simulink model "ex4"  (R2023b)
settings: Solver=FixedStepDiscrete  StartTime=0.0  StopTime=inf  FixedStep=0.0001  RelTol=1e-3
libraries: simulink_extras x4
settings Model: Creator=Andrei  LastModifiedBy=Andrei

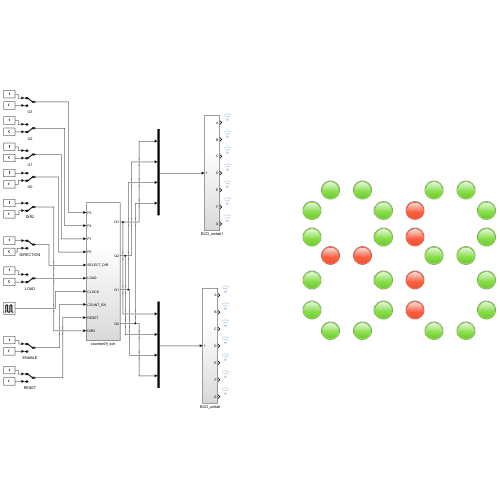
[thumbnail: Simulink's stored preview of the top-level diagram]
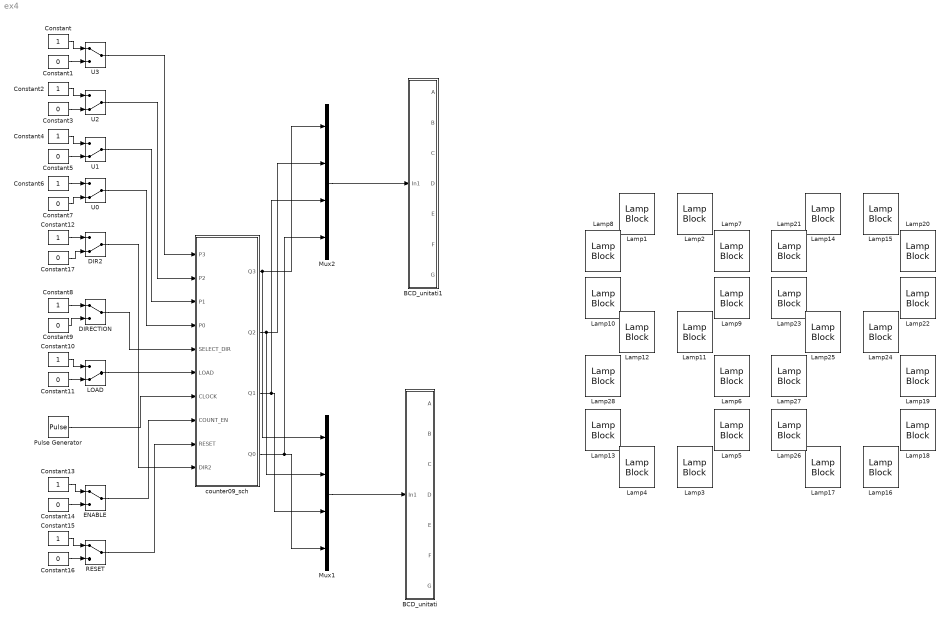
== system ex4 ==
  BCD_unitati : Subsystem
  BCD_unitati1 : Subsystem
  Constant{,2,4,6,8,10,12..13,15} (9 alike) : Constant
  Constant{1,3,5,7,9,11,14,16..17} (9 alike) : Constant  Value=0
  DIR2 : ManualSwitch  CurrentSetting=0
  DIRECTION : ManualSwitch
  ENABLE : ManualSwitch
  LOAD : ManualSwitch  CurrentSetting=0
  Lamp{1..28} (28 alike) : LampBlock  LabelPosition=Hide
  Mux1 : Mux
  Mux2 : Mux
  Pulse Generator : DiscretePulseGenerator  PulseType=Time based  Period=3  PulseWidth=5
  RESET : ManualSwitch
  U0 : ManualSwitch  CurrentSetting=0
  U1 : ManualSwitch  CurrentSetting=0
  U2 : ManualSwitch  CurrentSetting=0
  U3 : ManualSwitch
  counter09_sch : Subsystem
  wires:
  Constant11/1 -> LOAD/2
  Constant5/1 -> U1/2
  Mux1/1 -> BCD_unitati/1(In1)
  Constant4/1 -> U1/1
  Constant2/1 -> U2/1
  Constant13/1 -> ENABLE/1
  counter09_sch/3(Q1) -> Mux2/3, Mux1/3
  Constant6/1 -> U0/1
  counter09_sch/4(Q0) -> Mux1/4, Mux2/4
  counter09_sch/2(Q2) -> Mux1/2, Mux2/2
  Constant/1 -> U3/1
  Constant15/1 -> RESET/1
  RESET/1 -> counter09_sch/9(RESET)
  ENABLE/1 -> counter09_sch/8(COUNT_EN)
  LOAD/1 -> counter09_sch/6(LOAD)
  Pulse Generator/1 -> counter09_sch/7("CLOCK ")
  Constant10/1 -> LOAD/1
  DIRECTION/1 -> counter09_sch/5(SELECT_DIR)
  U1/1 -> counter09_sch/3(P1)
  Constant14/1 -> ENABLE/2
  U3/1 -> counter09_sch/1(P3)
  Constant3/1 -> U2/2
  Constant16/1 -> RESET/2
  U0/1 -> counter09_sch/4(P0)
  Constant17/1 -> DIR2/2
  Constant12/1 -> DIR2/1
  U2/1 -> counter09_sch/2(P2)
  Constant8/1 -> DIRECTION/1
  Constant1/1 -> U3/2
  DIR2/1 -> counter09_sch/10(DIR2)
  counter09_sch/1(Q3) -> Mux2/1, Mux1/1
  Mux2/1 -> BCD_unitati1/1(In1)
  Constant9/1 -> DIRECTION/2
  Constant7/1 -> U0/2

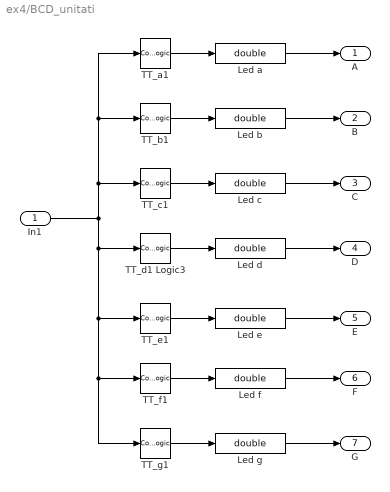
== system ex4/BCD_unitati ==
  In1 : Inport
  " TT_a1" : CombinatorialLogic  TruthTable=[1;0;1;1;0;1;1;1;1;1;0;0;0;0;0;0]
  " TT_c1" : CombinatorialLogic  TruthTable=[1;1;0;1;1;1;1;1;1;1;0;0;0;0;0;0]
  " TT_f1" : CombinatorialLogic  TruthTable=[1;0;0;0;1;1;1;0;1;1;0;0;0;0;0;0]
  " TT_g1" : CombinatorialLogic  TruthTable=[0;0;1;1;1;1;1;0;1;1;0;0;0;0;0;0]
  Led a : DataTypeConversion  OutDataTypeStr=double  SaturateOnIntegerOverflow=off  RndMeth=Floor
  Led b : DataTypeConversion  OutDataTypeStr=double  SaturateOnIntegerOverflow=off  RndMeth=Floor
  Led c : DataTypeConversion  OutDataTypeStr=double  SaturateOnIntegerOverflow=off  RndMeth=Floor
  Led d : DataTypeConversion  OutDataTypeStr=double  SaturateOnIntegerOverflow=off  RndMeth=Floor
  Led e : DataTypeConversion  OutDataTypeStr=double  SaturateOnIntegerOverflow=off  RndMeth=Floor
  Led f : DataTypeConversion  OutDataTypeStr=double  SaturateOnIntegerOverflow=off  RndMeth=Floor
  Led g : DataTypeConversion  OutDataTypeStr=double  SaturateOnIntegerOverflow=off  RndMeth=Floor
  TT_b1 : CombinatorialLogic  TruthTable=[1;1;1;1;1;0;0;1;1;1;0;0;0;0;0;0]
  TT_d1 Logic3 : CombinatorialLogic  TruthTable=[1;0;1;1;0;1;1;0;1;1;0;0;0;0;0;0]
  TT_e1 : CombinatorialLogic  TruthTable=[1;0;1;0;0;0;1;0;1;0;0;0;0;0;0;0]
  A : Outport
  B : Outport  Port=2
  C : Outport  Port=3
  D : Outport  Port=4
  E : Outport  Port=5
  F : Outport  Port=6
  G : Outport  Port=7
  wires:
  Led a/1 -> A/1
  " TT_f1"/1 -> Led f/1
  TT_d1 Logic3/1 -> Led d/1
  In1/1 -> " TT_c1"/1, TT_b1/1, " TT_a1"/1, TT_d1 Logic3/1, TT_e1/1, " TT_f1"/1, " TT_g1"/1
  " TT_g1"/1 -> Led g/1
  TT_e1/1 -> Led e/1
  " TT_c1"/1 -> Led c/1
  " TT_a1"/1 -> Led a/1
  TT_b1/1 -> Led b/1
  Led b/1 -> B/1
  Led d/1 -> D/1
  Led c/1 -> C/1
  Led e/1 -> E/1
  Led f/1 -> F/1
  Led g/1 -> G/1

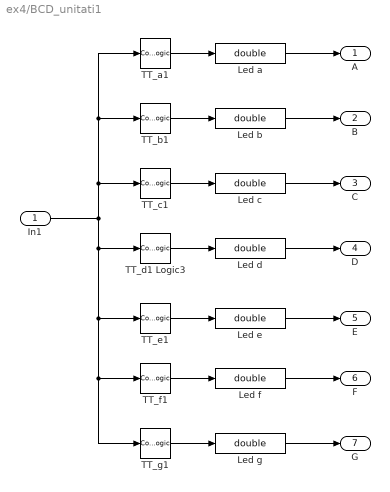
== system ex4/BCD_unitati1 ==
  In1 : Inport
  " TT_a1" : CombinatorialLogic  TruthTable=[1;1;1;1;1;1;1;1;1;1;0;0;0;0;0;0]
  " TT_c1" : CombinatorialLogic  TruthTable=[1;1;1;1;1;1;1;1;1;1;1;1;1;1;1;1]
  " TT_f1" : CombinatorialLogic  TruthTable=[1;1;1;1;1;1;1;1;1;1;0;0;0;0;0;0]
  " TT_g1" : CombinatorialLogic  TruthTable=[0;0;0;0;0;0;0;0;0;0;0;0;0;0;0;0]
  Led a : DataTypeConversion  OutDataTypeStr=double  SaturateOnIntegerOverflow=off  RndMeth=Floor
  Led b : DataTypeConversion  OutDataTypeStr=double  SaturateOnIntegerOverflow=off  RndMeth=Floor
  Led c : DataTypeConversion  OutDataTypeStr=double  SaturateOnIntegerOverflow=off  RndMeth=Floor
  Led d : DataTypeConversion  OutDataTypeStr=double  SaturateOnIntegerOverflow=off  RndMeth=Floor
  Led e : DataTypeConversion  OutDataTypeStr=double  SaturateOnIntegerOverflow=off  RndMeth=Floor
  Led f : DataTypeConversion  OutDataTypeStr=double  SaturateOnIntegerOverflow=off  RndMeth=Floor
  Led g : DataTypeConversion  OutDataTypeStr=double  SaturateOnIntegerOverflow=off  RndMeth=Floor
  TT_b1 : CombinatorialLogic  TruthTable=[1;1;1;1;1;1;1;1;1;1;1;1;1;1;1;1]
  TT_d1 Logic3 : CombinatorialLogic  TruthTable=[1;1;1;1;1;1;1;1;1;1;0;0;0;0;0;0]
  TT_e1 : CombinatorialLogic  TruthTable=[1;1;1;1;1;1;1;1;1;1;0;0;0;0;0;0]
  A : Outport
  B : Outport  Port=2
  C : Outport  Port=3
  D : Outport  Port=4
  E : Outport  Port=5
  F : Outport  Port=6
  G : Outport  Port=7
  wires:
  Led a/1 -> A/1
  " TT_f1"/1 -> Led f/1
  TT_d1 Logic3/1 -> Led d/1
  In1/1 -> " TT_c1"/1, TT_b1/1, " TT_a1"/1, TT_d1 Logic3/1, TT_e1/1, " TT_f1"/1, " TT_g1"/1
  " TT_g1"/1 -> Led g/1
  TT_e1/1 -> Led e/1
  " TT_c1"/1 -> Led c/1
  " TT_a1"/1 -> Led a/1
  TT_b1/1 -> Led b/1
  Led b/1 -> B/1
  Led d/1 -> D/1
  Led c/1 -> C/1
  Led e/1 -> E/1
  Led f/1 -> F/1
  Led g/1 -> G/1

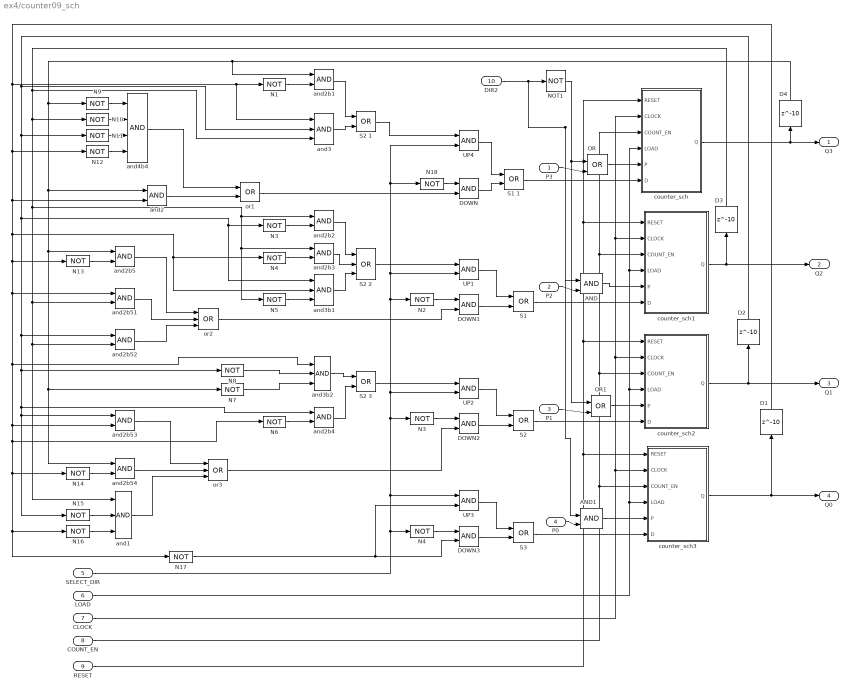
== system ex4/counter09_sch ==
  P3 : Inport
  P2 : Inport  Port=2
  P1 : Inport  Port=3
  P0 : Inport  Port=4
  SELECT_DIR : Inport  Port=5
  LOAD : Inport  Port=6
  "CLOCK " : Inport  Port=7
  COUNT_EN : Inport  Port=8
  RESET : Inport  Port=9
  DIR2 : Inport  Port=10
  AND : Logic  IconShape=distinctive  AllPortsSameDT=off  OutDataTypeStr=boolean
  AND1 : Logic  IconShape=distinctive  AllPortsSameDT=off  OutDataTypeStr=boolean
  D{1..4} (4 alike) : Delay  DelayLength=10  InitialCondition=1
  DOWN{,1..3} (4 alike) : Logic  AllPortsSameDT=off  OutDataTypeStr=boolean
  N{1..18} (18 alike) : Logic  Operator=NOT  AllPortsSameDT=off  OutDataTypeStr=boolean
  "N3 " : Logic  Operator=NOT  AllPortsSameDT=off  OutDataTypeStr=boolean
  "N4 " : Logic  Operator=NOT  AllPortsSameDT=off  OutDataTypeStr=boolean
  NOT1 : Logic  Operator=NOT  IconShape=distinctive  AllPortsSameDT=off  OutDataTypeStr=boolean
  OR : Logic  Operator=OR  IconShape=distinctive  AllPortsSameDT=off  OutDataTypeStr=boolean
  OR1 : Logic  Operator=OR  IconShape=distinctive  AllPortsSameDT=off  OutDataTypeStr=boolean
  "S1 " : Logic  Operator=OR  AllPortsSameDT=off  OutDataTypeStr=boolean
  S1 1 : Logic  Operator=OR  AllPortsSameDT=off  OutDataTypeStr=boolean
  "S2 " : Logic  Operator=OR  AllPortsSameDT=off  OutDataTypeStr=boolean
  S2 1 : Logic  Operator=OR  AllPortsSameDT=off  OutDataTypeStr=boolean
  S2 2 : Logic  Operator=OR  Inputs=3  AllPortsSameDT=off  OutDataTypeStr=boolean
  S2 3 : Logic  Operator=OR  AllPortsSameDT=off  OutDataTypeStr=boolean
  "S3 " : Logic  Operator=OR  AllPortsSameDT=off  OutDataTypeStr=boolean
  UP{1..4} (4 alike) : Logic  AllPortsSameDT=off  OutDataTypeStr=boolean
  and1 : Logic  Inputs=3  AllPortsSameDT=off  OutDataTypeStr=boolean
  and2 : Logic  AllPortsSameDT=off  OutDataTypeStr=boolean
  and2b{1..5,51..54} (9 alike) : Logic  AllPortsSameDT=off  OutDataTypeStr=boolean
  and3 : Logic  Inputs=3  AllPortsSameDT=off  OutDataTypeStr=boolean
  and3b1 : Logic  Inputs=3  AllPortsSameDT=off  OutDataTypeStr=boolean
  and3b2 : Logic  Inputs=3  AllPortsSameDT=off  OutDataTypeStr=boolean
  and4b4 : Logic  Inputs=4  AllPortsSameDT=off  OutDataTypeStr=boolean
  counter_sch : Subsystem
  counter_sch1 : Subsystem
  counter_sch2 : Subsystem
  counter_sch3 : Subsystem
  or1 : Logic  Operator=OR  AllPortsSameDT=off  OutDataTypeStr=boolean
  or2 : Logic  Operator=OR  Inputs=3  AllPortsSameDT=off  OutDataTypeStr=boolean
  or3 : Logic  Operator=OR  Inputs=3  AllPortsSameDT=off  OutDataTypeStr=boolean
  Q3 : Outport
  Q2 : Outport  Port=2
  Q1 : Outport  Port=3
  Q0 : Outport  Port=4
  wires:
  N11/1 -> and4b4/3
  and2b53/1 -> or3/1
  and2/1 -> or1/2
  or3/1 -> DOWN2/2
  and2b5/1 -> or2/1
  and2b3/1 -> S2 2/2
  and2b54/1 -> or3/2
  and3b1/1 -> S2 2/3
  N6/1 -> and2b4/2
  N3/1 -> and2b2/2
  D4/1 -> and2b1/1, and2/1, and2b5/1, N7/1, and2b54/1, N9/1
  and3b2/1 -> S2 3/1
  N8/1 -> and3b2/2
  N7/1 -> and3b2/3
  and4b4/1 -> or1/1
  and2b51/1 -> or2/2
  N16/1 -> and1/3
  and2b52/1 -> or2/3
  N14/1 -> and2b54/2
  N4/1 -> and2b3/2
  N12/1 -> and4b4/4
  N13/1 -> and2b5/2
  N1/1 -> and2b1/2
  and2b2/1 -> S2 2/1
  and1/1 -> or3/3
  D2/1 -> and2b52/1, N8/1, and2b4/1, N15/1, and2b53/1, N3/1, and3b1/1, N11/1, and3/2
  or2/1 -> DOWN1/2
  and2b4/1 -> S2 3/2
  N15/1 -> and1/2
  N17/1 -> UP3/2, DOWN3/2
  N9/1 -> and4b4/1
  N5/1 -> and3b1/3
  D3/1 -> and2b2/1, and2b3/1, N5/1, and2b51/2, and2b52/2, and1/1, N10/1, and3/3
  D1/1 -> and2/2, N4/1, and3b1/2, N13/1, and2b51/1, and3b2/1, N6/1, N14/1, N16/1, N17/1, and2b53/2, N12/1, and3/1, N1/1
  "S1 "/1 -> counter_sch1/6(D)
  "S2 "/1 -> counter_sch2/6(D)
  "S3 "/1 -> counter_sch3/6(D)
  N10/1 -> and4b4/2
  "CLOCK "/1 -> counter_sch/2(CLOCK), counter_sch1/2(CLOCK), counter_sch2/2(CLOCK), counter_sch3/2(CLOCK)
  LOAD/1 -> counter_sch/4(LOAD), counter_sch1/4(LOAD), counter_sch2/4(LOAD), counter_sch3/4(LOAD)
  COUNT_EN/1 -> counter_sch/3(COUNT_EN), counter_sch1/3(COUNT_EN), counter_sch2/3(COUNT_EN), counter_sch3/3(COUNT_EN)
  RESET/1 -> counter_sch/1(RESET), counter_sch1/1(RESET), counter_sch2/1(RESET), counter_sch3/1(RESET)
  DOWN1/1 -> "S1 "/2
  UP1/1 -> "S1 "/1
  "N3 "/1 -> DOWN2/1
  DOWN3/1 -> "S3 "/2
  UP3/1 -> "S3 "/1
  UP2/1 -> "S2 "/1
  DOWN2/1 -> "S2 "/2
  N2/1 -> DOWN1/1
  "N4 "/1 -> DOWN3/1
  S2 2/1 -> UP1/1
  S2 3/1 -> UP2/1
  and3/1 -> S2 1/2
  SELECT_DIR/1 -> "N4 "/1, UP3/1, "N3 "/1, UP2/2, N2/1, UP4/2, N18/1, UP1/2
  and2b1/1 -> S2 1/1
  counter_sch3/1(Q) -> Q0/1, D1/1
  counter_sch2/1(Q) -> Q1/1, D2/1
  counter_sch1/1(Q) -> Q2/1, D3/1
  counter_sch/1(Q) -> Q3/1, D4/1
  UP4/1 -> S1 1/1
  DOWN/1 -> S1 1/2
  N18/1 -> DOWN/1
  S2 1/1 -> UP4/1
  or1/1 -> DOWN/2
  S1 1/1 -> counter_sch/6(D)
  DIR2/1 -> AND/1, AND1/1, NOT1/1
  NOT1/1 -> OR1/1, OR/1
  P3/1 -> OR/2
  OR/1 -> counter_sch/5(P)
  P1/1 -> OR1/2
  OR1/1 -> counter_sch2/5(P)
  P0/1 -> AND1/2
  AND1/1 -> counter_sch3/5(P)
  P2/1 -> AND/2
  AND/1 -> counter_sch1/5(P)

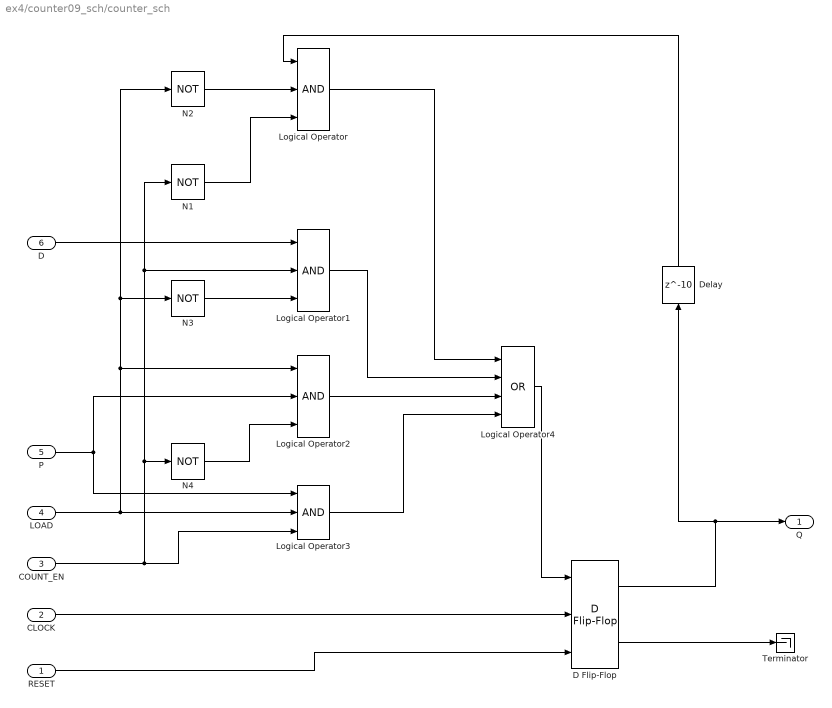
== system ex4/counter09_sch/counter_sch ==
  RESET : Inport
  CLOCK : Inport  Port=2
  COUNT_EN : Inport  Port=3
  LOAD : Inport  Port=4
  P : Inport  Port=5
  D : Inport  Port=6
  D Flip-Flop : simulink_extras/Flip Flops/D Flip-Flop
  Delay : Delay  DelayLength=10  InitialCondition=1
  Logical Operator{,1..3} (4 alike) : Logic  Inputs=3  AllPortsSameDT=off  OutDataTypeStr=boolean
  Logical Operator4 : Logic  Operator=OR  Inputs=4  AllPortsSameDT=off  OutDataTypeStr=boolean
  N{1..4} (4 alike) : Logic  Operator=NOT  Inputs=3  AllPortsSameDT=off  OutDataTypeStr=boolean
  Terminator : Terminator
  Q : Outport
  wires:
  D Flip-Flop/2 -> Terminator/1
  P/1 -> Logical Operator3/1, Logical Operator2/2
  Logical Operator1/1 -> Logical Operator4/2
  Logical Operator/1 -> Logical Operator4/1
  Delay/1 -> Logical Operator/1
  Logical Operator3/1 -> Logical Operator4/4
  CLOCK/1 -> D Flip-Flop/2
  D/1 -> Logical Operator1/1
  N3/1 -> Logical Operator1/3
  D Flip-Flop/1 -> Q/1, Delay/1
  N4/1 -> Logical Operator2/3
  LOAD/1 -> Logical Operator3/2, Logical Operator2/1, N3/1, N2/1
  RESET/1 -> D Flip-Flop/3
  N1/1 -> Logical Operator/3
  Logical Operator4/1 -> D Flip-Flop/1
  Logical Operator2/1 -> Logical Operator4/3
  COUNT_EN/1 -> Logical Operator3/3, N4/1, Logical Operator1/2, N1/1
  N2/1 -> Logical Operator/2

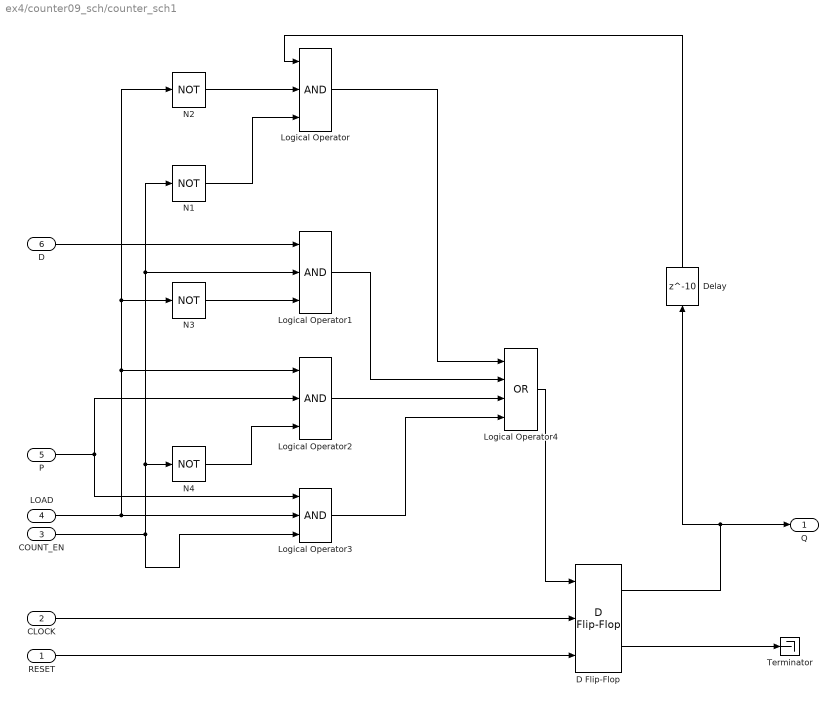
== system ex4/counter09_sch/counter_sch1 ==
  RESET : Inport
  CLOCK : Inport  Port=2
  COUNT_EN : Inport  Port=3
  LOAD : Inport  Port=4
  P : Inport  Port=5
  D : Inport  Port=6
  D Flip-Flop : simulink_extras/Flip Flops/D Flip-Flop
  Delay : Delay  DelayLength=10  InitialCondition=1
  Logical Operator{,1..3} (4 alike) : Logic  Inputs=3  AllPortsSameDT=off  OutDataTypeStr=boolean
  Logical Operator4 : Logic  Operator=OR  Inputs=4  AllPortsSameDT=off  OutDataTypeStr=boolean
  N{1..4} (4 alike) : Logic  Operator=NOT  Inputs=3  AllPortsSameDT=off  OutDataTypeStr=boolean
  Terminator : Terminator
  Q : Outport
  wires:
  D Flip-Flop/2 -> Terminator/1
  P/1 -> Logical Operator3/1, Logical Operator2/2
  Logical Operator1/1 -> Logical Operator4/2
  Logical Operator/1 -> Logical Operator4/1
  Delay/1 -> Logical Operator/1
  Logical Operator3/1 -> Logical Operator4/4
  CLOCK/1 -> D Flip-Flop/2
  D/1 -> Logical Operator1/1
  N3/1 -> Logical Operator1/3
  D Flip-Flop/1 -> Q/1, Delay/1
  N4/1 -> Logical Operator2/3
  LOAD/1 -> Logical Operator3/2, Logical Operator2/1, N3/1, N2/1
  RESET/1 -> D Flip-Flop/3
  N1/1 -> Logical Operator/3
  Logical Operator4/1 -> D Flip-Flop/1
  Logical Operator2/1 -> Logical Operator4/3
  COUNT_EN/1 -> Logical Operator3/3, N4/1, Logical Operator1/2, N1/1
  N2/1 -> Logical Operator/2

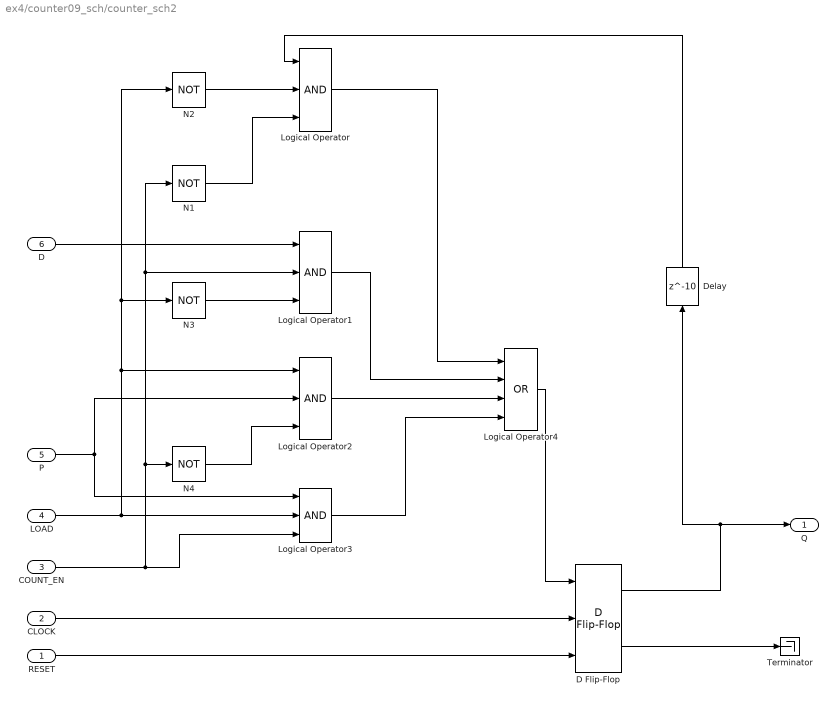
== system ex4/counter09_sch/counter_sch2 ==
  RESET : Inport
  CLOCK : Inport  Port=2
  COUNT_EN : Inport  Port=3
  LOAD : Inport  Port=4
  P : Inport  Port=5
  D : Inport  Port=6
  D Flip-Flop : simulink_extras/Flip Flops/D Flip-Flop
  Delay : Delay  DelayLength=10  InitialCondition=1
  Logical Operator{,1..3} (4 alike) : Logic  Inputs=3  AllPortsSameDT=off  OutDataTypeStr=boolean
  Logical Operator4 : Logic  Operator=OR  Inputs=4  AllPortsSameDT=off  OutDataTypeStr=boolean
  N{1..4} (4 alike) : Logic  Operator=NOT  Inputs=3  AllPortsSameDT=off  OutDataTypeStr=boolean
  Terminator : Terminator
  Q : Outport
  wires:
  D Flip-Flop/2 -> Terminator/1
  P/1 -> Logical Operator3/1, Logical Operator2/2
  Logical Operator1/1 -> Logical Operator4/2
  Logical Operator/1 -> Logical Operator4/1
  Delay/1 -> Logical Operator/1
  Logical Operator3/1 -> Logical Operator4/4
  CLOCK/1 -> D Flip-Flop/2
  D/1 -> Logical Operator1/1
  N3/1 -> Logical Operator1/3
  D Flip-Flop/1 -> Q/1, Delay/1
  N4/1 -> Logical Operator2/3
  LOAD/1 -> Logical Operator3/2, Logical Operator2/1, N3/1, N2/1
  RESET/1 -> D Flip-Flop/3
  N1/1 -> Logical Operator/3
  Logical Operator4/1 -> D Flip-Flop/1
  Logical Operator2/1 -> Logical Operator4/3
  COUNT_EN/1 -> Logical Operator3/3, N4/1, Logical Operator1/2, N1/1
  N2/1 -> Logical Operator/2

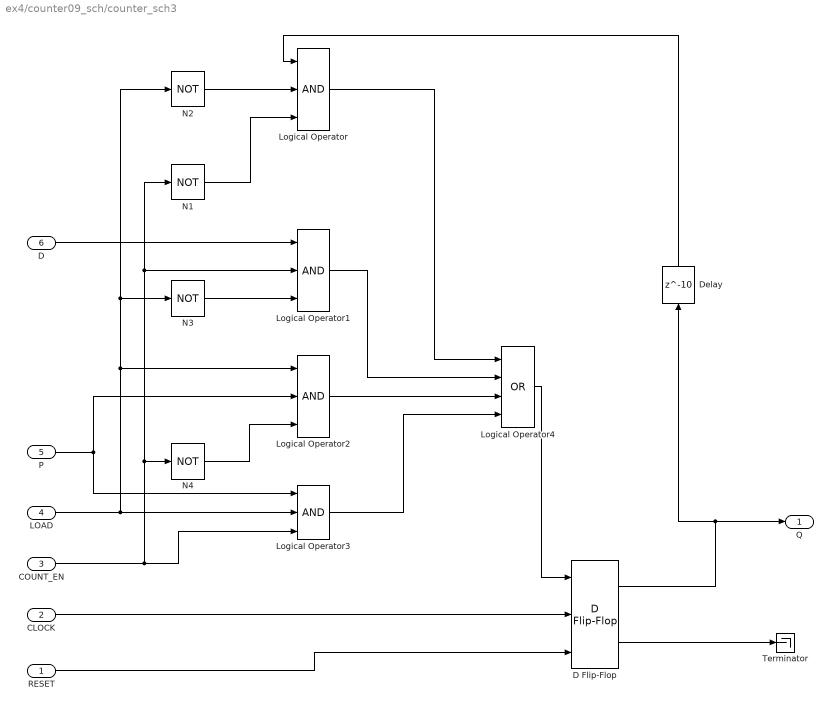
== system ex4/counter09_sch/counter_sch3 ==
  RESET : Inport
  CLOCK : Inport  Port=2
  COUNT_EN : Inport  Port=3
  LOAD : Inport  Port=4
  P : Inport  Port=5
  D : Inport  Port=6
  D Flip-Flop : simulink_extras/Flip Flops/D Flip-Flop
  Delay : Delay  DelayLength=10  InitialCondition=1
  Logical Operator{,1..3} (4 alike) : Logic  Inputs=3  AllPortsSameDT=off  OutDataTypeStr=boolean
  Logical Operator4 : Logic  Operator=OR  Inputs=4  AllPortsSameDT=off  OutDataTypeStr=boolean
  N{1..4} (4 alike) : Logic  Operator=NOT  Inputs=3  AllPortsSameDT=off  OutDataTypeStr=boolean
  Terminator : Terminator
  Q : Outport
  wires:
  D Flip-Flop/2 -> Terminator/1
  P/1 -> Logical Operator3/1, Logical Operator2/2
  Logical Operator1/1 -> Logical Operator4/2
  Logical Operator/1 -> Logical Operator4/1
  Delay/1 -> Logical Operator/1
  Logical Operator3/1 -> Logical Operator4/4
  CLOCK/1 -> D Flip-Flop/2
  D/1 -> Logical Operator1/1
  N3/1 -> Logical Operator1/3
  D Flip-Flop/1 -> Q/1, Delay/1
  N4/1 -> Logical Operator2/3
  LOAD/1 -> Logical Operator3/2, Logical Operator2/1, N3/1, N2/1
  RESET/1 -> D Flip-Flop/3
  N1/1 -> Logical Operator/3
  Logical Operator4/1 -> D Flip-Flop/1
  Logical Operator2/1 -> Logical Operator4/3
  COUNT_EN/1 -> Logical Operator3/3, N4/1, Logical Operator1/2, N1/1
  N2/1 -> Logical Operator/2
